simulink model "SG__REF_O"  (R2022b)
settings: Solver=FixedStepAuto  StartTime=0.0  StopTime=Inf  RelTol=1e-3  EnableMultiTasking=on
model workspace (MAT data in the model file):
  N_trig = Simulink.Parameter
  N_trig.Value = 4
  N_trig.Description = 'number of samples for triggered pulse for recording'
  N_trig.DataType = 'auto'
  N_trig.Complexity = 'real'
  N_trig.Dimensions = [1 1]
  a_1 = Simulink.Parameter
  a_1.Value = [1 1 1]
  a_1.DataType = 'auto'
  a_1.Complexity = 'real'
  a_1.Dimensions = [1 3]
  b_1 = Simulink.Parameter
  b_1.Value = [0.5 0.5 0.5]
  b_1.DataType = 'auto'
  b_1.Complexity = 'real'
  b_1.Dimensions = [1 3]
  enable_source = Simulink.Parameter
  enable_source.Value = 0
  enable_source.DataType = 'boolean'
  enable_source.Complexity = 'real'
  enable_source.Dimensions = [1 1]
  freq_fin = Simulink.Parameter
  freq_fin.Value = 1200
  freq_fin.DataType = 'auto'
  freq_fin.Complexity = 'real'
  freq_fin.Dimensions = [1 1]
  freq_ini = Simulink.Parameter
  freq_ini.Value = 150
  freq_ini.DataType = 'auto'
  freq_ini.Complexity = 'real'
  freq_ini.Dimensions = [1 1]
  k_1 = Simulink.Parameter
  k_1.Value = [0 0 0]
  k_1.DataType = 'auto'
  k_1.Complexity = 'real'
  k_1.Dimensions = [1 3]
  rec = Simulink.Parameter
  rec.Value = 0
  rec.DataType = 'boolean'
  rec.Complexity = 'real'
  rec.Dimensions = [1 1]
  src_select = Simulink.Parameter
  src_select.Value = 0
  src_select.DataType = 'auto'
  src_select.Complexity = 'real'
  src_select.Dimensions = [1 1]
  sweep_gain = Simulink.Parameter
  sweep_gain.Value = 0.02
  sweep_gain.DataType = 'auto'
  sweep_gain.Complexity = 'real'
  sweep_gain.Dimensions = [1 1]
  tmax = Simulink.Parameter
  tmax.Value = 10
  tmax.DataType = 'auto'
  tmax.Complexity = 'real'
  tmax.Dimensions = [1 1]
  ts_rec = Simulink.Parameter
  ts_rec.Value = 0.0001
  ts_rec.DataType = 'auto'
  ts_rec.Complexity = 'real'
  ts_rec.Dimensions = [1 1]
undefined symbols (not defined in the file or in its folder): Ended, Single
libraries: speedgoatlib_IO135 x2, speedgoatlib_IO104 x2, simulink x1, slrealtimetgmanagement x1
settings Model: SimulationMode=external  DataflowThreadingImplementation=Pthreads  Creator=padlewsk  LastModifiedBy=padlewsk
settings SolverCC: ConcurrentTasks=on  AlgebraicLoopSolver=TrustRegion  PositivePriorityOrder=on  AutoInsertRateTranBlk=on
settings DataIOCC: SaveFormat=StructureWithTime
settings OptimizationCC: GainParamInheritBuiltInType=on  RollThreshold=9  EfficientFloat2IntCast=on  SimCompilerOptimization=on
settings DebuggingCC: TasksWithSamePriorityMsg=none  UnconnectedInputMsg=warning  UnconnectedOutputMsg=warning  UnconnectedLineMsg=warning
settings HardwareCC: ProdBitPerLong=64  ProdLongLongMode=on  ProdHWDeviceType=Intel->x86-64 (Linux 64)
settings ModelReferenceCC: EnableRefExpFcnMdlSchedulingChecks=on  ModelReferenceNumInstancesAllowed=Single
settings RTWCC: Description=Simulink Real-Time  SystemTargetFile=slrealtime.tlc  TemplateMakefile=slrealtime_default_tmf  Toolchain=Simulink Real-Time Toolchain  BuildConfiguration=Faster Runs  CodeExecutionProfiling=on  TargetLang=C++

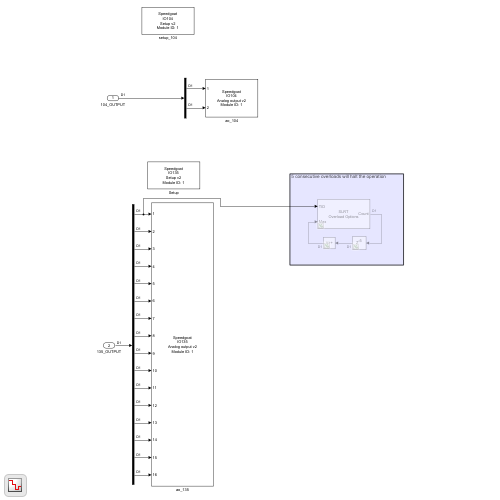
[thumbnail: Simulink's stored preview of the top-level diagram]
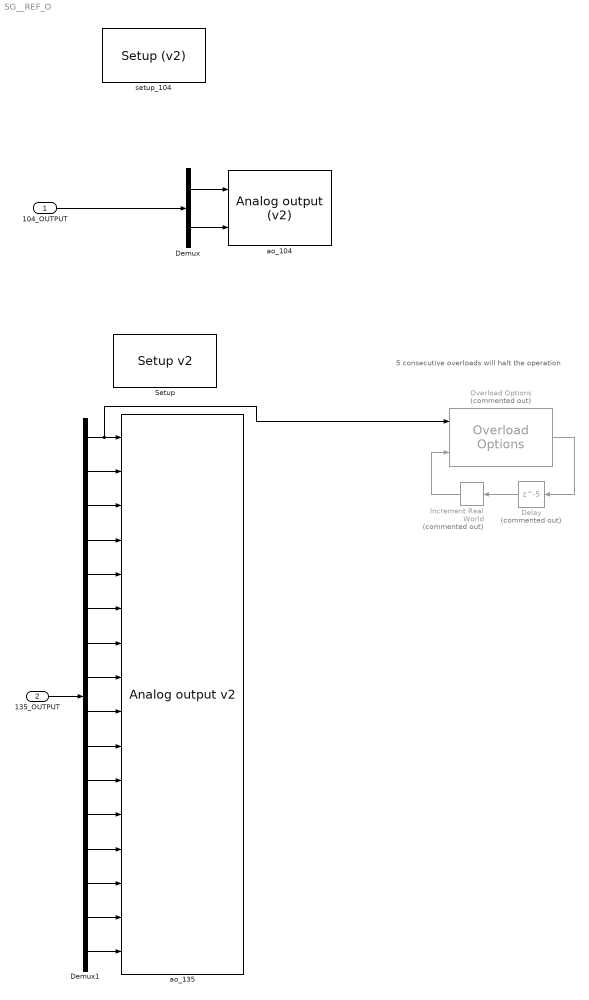
== system SG__REF_O ==
  note: 5 consecutive overloads will halt the operation
  104_OUTPUT : Inport
  135_OUTPUT : Inport  Port=2
  Delay : Delay  Commented=on  DelayLength=5
  Demux : Demux  Outputs=2
  Demux1 : Demux  Outputs=16
  Increment Real World : simulink/Additional Math & Discrete/Additional Math: Increment - Decrement/Increment Real World  Commented=on
  Overload Options : slrealtimetgmanagement/Overload Options  Commented=on  startupDur=1  startupDurSrc=Tunable Parameter  maxOverload=0  maxOverloadSrc=Input Port  TETFlag=off
  Setup : speedgoatlib_IO135/Setup v2   parPciSlot=-1  parModuleId=1  parInterModuleSync=None  parConvClockBaseRate=60MHz  parConvClock1Divider=20000  parConvClock2Divider=20000  parFrameTriggerEnable=off  parFrameTriggerDivider=10  parConvClock1BaseRate=3  parConvClock2BaseRate=3  parFrameTriggerClock=1  parAdcChannels=[1:32]  parAdcRange1=+-5V  parAdcRange2=+-5V  parAdcRange3=+-5V  parAdcRange4=+-5V  parAdcVoltageRange=[1 1 1 1]  parAdcOversampling1=None  parAdcOversampling2=None  parAdcOversampling3=None  parAdcOversampling4=None  parAdcOversamplRate=[1 1 1 1]  parAdcAutoCorrection=on  parAdcContSampling=off  parAdcDmaEnable=off  parAdcDmaClock=Clock 1  parAdcFrameSize_=100  parAdcSampleTime_=-1  parAdcActiveDmaDevices=[1 1 1 1]  parAdcFrameTriggerEnable=0  parAdcFrameSize=100  parAdcSampleTime=0.0333333333333333  parDacChannels=[1:16]  parDacInitValues=0  parDacReset=1  parDacRange1=+-10V  parDacRange2=+-10V  parDacRange3=+-10V  parDacRange4=+-10V  parDacRange5=+-10V  parDacRange6=+-10V  parDacRange7=+-10V  parDacRange8=+-10V  parDacRange9=+-10V  parDacRange10=+-10V  parDacRange11=+-10V  parDacRange12=+-10V  parDacRange13=+-10V  parDacRange14=+-10V  parDacRange15=+-10V  parDacRange16=+-10V  parDacVoltageRange=[5 5 5 5 5 5 5 5 5 5 5 5 5 5 5 5]  parDacAutoCorrection=on  parDacSyncOut=off  parDacDmaEnable=off  parDacDmaLatency=Until next frame  parDacDmaClock=Clock 1  parDacFrameSize_=100  parDacSampleTime_=-1  parDacActiveDmaDevices=[1 1 1 1]  parDacFrameTriggerEnable=0  parDacFrameSize=100  parDacSampleTime=0.0333333333333333  parDoChannels=[]  parDoInitValues=0  parDoReset=1  parDiChannels=[]  parDiDebounceEnable=off  parDiDebounceTime=0  parDiDebounceValue=0  parDioPullRefFront=Pull-up 3.3V  parDioPullRefRear=Floating
      settings: SourceProductName=Simulink Real-Time: Speedgoat I/O Blockset
  ao_104 : speedgoatlib_IO104/Analog output (v2)   parModuleId=1  parTs=ts  parPciSlot=-1  parDaSimultaneous=on  parDaChannels=[1,2]  parDaChannelsSorted=[1,2]  parDaInitValue=[0,0]  parDaReset=[1,1]  parDaRange=+-10V  parDaFrameSize=1  parDaUseTrigger=off  parDaClockInitiator=Initiator  parDaSampleTime=9.920634921e-07  parTriggerInitiator=Initiator  parTriggerRate=4.161015625e-01  parAdBlockPresent=0
      settings: SourceProductName=Simulink Real-Time: Speedgoat I/O Blockset
  ao_135 : speedgoatlib_IO135/Analog output v2   parModuleId=1  parSampleTime=ts  parPciSlot=-1  parDacChannels=[1 2 3 4 5 6 7 8 9 10 11 12 13 14 15 16]  parDacVoltageRange=[5 5 5 5 5 5 5 5 5 5 5 5 5 5 5 5]  parDacInitValues=[0 0 0 0 0 0 0 0 0 0 0 0 0 0 0 0]  parDacReset=[1 1 1 1 1 1 1 1 1 1 1 1 1 1 1 1]  parDacSyncOut=0  parDacDmaEnable=0  parDacActiveDmaDevices=[1 1 1 1]  parDacDmaLatency=2  parDacFrameSize=100
      settings: SourceProductName=Simulink Real-Time: Speedgoat I/O Blockset
  setup_104 : speedgoatlib_IO104/Setup (v2)   parPciSlot=-1  parModuleId=1  parTriggerInitiator=Initiator  parTriggerRate=4.161015625e-01  parCalibrate=off  parAdChannels=[1:8]  parAdRange1=+-2.5V  parAdRange2=+-2.5V  parAdCoupling=Single-Ended  parAdUseTrigger=off  parAdFrameSize=1  parAdClockInitiator=Initiator  parAdSampleTime=9.920634921e-07  parDaSimultaneous=on  parDaChannels=[1:2]  parDaChannelsSorted=[1,2]  parDaInitValue=[0]  parDaReset=[1]  parDaRange=+-10V  parDaUseTrigger=off  parDaFrameSize=1  parDaClockInitiator=Initiator  parDaSampleTime=9.920634921e-07  parDioByte0Dir=Outputs  parDioByte1Dir=Inputs  parDoChannels=[]  parDoInitValues=[0]  parDoReset=[1]  parDiChannels=[]
      settings: SourceProductName=Simulink Real-Time: Speedgoat I/O Blockset
  wires:
  Demux/1 -> ao_104/1
  Demux/2 -> ao_104/2
  104_OUTPUT/1 -> Demux/1
  Demux1/7 -> ao_135/7
  Demux1/1 -> Overload Options/1, ao_135/1
  Demux1/6 -> ao_135/6
  Demux1/2 -> ao_135/2
  Demux1/3 -> ao_135/3
  135_OUTPUT/1 -> Demux1/1
  Demux1/16 -> ao_135/16
  Demux1/4 -> ao_135/4
  Demux1/10 -> ao_135/10
  Demux1/14 -> ao_135/14
  Demux1/13 -> ao_135/13
  Demux1/15 -> ao_135/15
  Demux1/11 -> ao_135/11
  Demux1/12 -> ao_135/12
  Demux1/9 -> ao_135/9
  Demux1/8 -> ao_135/8
  Demux1/5 -> ao_135/5
  Overload Options/1 -> Delay/1
  Increment Real World/1 -> Overload Options/2
  Delay/1 -> Increment Real World/1
